simulink model "gain"  (R2024b)
settings: Solver=VariableStepAuto  StartTime=0.0  StopTime=10.0  RelTol=1e-3
settings Model: Creator=ben  LastModifiedBy=ben

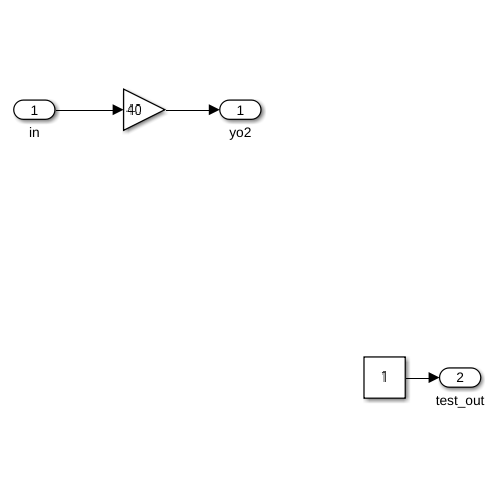
[thumbnail: Simulink's stored preview of the top-level diagram]
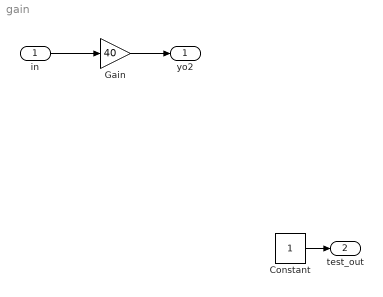
== system gain ==
  in : Inport
  Constant : Constant
  Gain : Gain  Gain=40
  yo2 : Outport
  test_out : Outport  Port=2
  wires:
  in/1 -> Gain/1
  Gain/1 -> yo2/1
  Constant/1 -> test_out/1
